simulink model "etasetget256Discretized2"  (R2015b)
settings: Solver=FixedStepAuto  StartTime=0.0  StopTime=inf  FixedStep=0.05  RelTol=1e-3
undefined symbols (not defined in the file or in its folder): X, Y, Z
libraries: robotlib x5
settings Model: Creator=einar  LastModifiedBy=einar
settings OptimizationCC: OptimizeModelRefInitCode=on  LifeSpan=Inf  MaxStackSize=64
settings HardwareCC: ProdBitPerPointer=32  ProdLargestAtomicFloat=None  ProdIntDivRoundTo=Undefined  ProdEndianess=Unspecified  ProdWordSize=32  ProdHWDeviceType=Generic->Unspecified (assume 32-bit Generic)
settings RTWCC: SystemTargetFile=ert.tlc  TemplateMakefile=ert_default_tmf  Description=Embedded Coder  Toolchain=Catkin  TargetLang=C++
settings CodeAppCC: IgnoreCustomStorageClasses=off
settings ERTTargetCC: SupportContinuousTime=on  SupportVariableSizeSignals=on

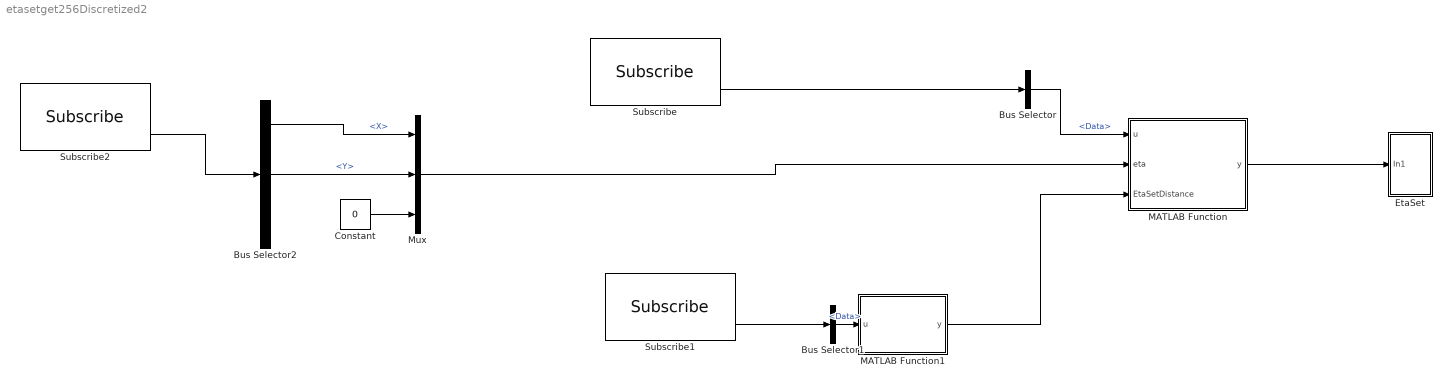
== system etasetget256Discretized2 ==
  Bus Selector : BusSelector  OutputSignals=Data
  Bus Selector1 : BusSelector  OutputSignals=Data
  Bus Selector2 : BusSelector  OutputSignals=X,Y,Z
  Constant : Constant  Value=0
  EtaSet : Subsystem
  MATLAB Function : MATLAB Function  TreatAsAtomicUnit=on
  MATLAB Function1 : MATLAB Function  TreatAsAtomicUnit=on
  Mux : Mux  Inputs=3
  Subscribe : robotlib/Subscribe  SourceLibraryInfo=This block requires Robotics System Toolbox  topicSource=Select from ROS network  topic=/EtaSetList  messageType=std_msgs/Float32MultiArray  sampleTime=-1  messageQueueLength=1
  Subscribe1 : robotlib/Subscribe  SourceLibraryInfo=This block requires Robotics System Toolbox  topicSource=Specify your own  topic=/EtaSetDistance  messageType=std_msgs/Float64  sampleTime=-1  messageQueueLength=1
  Subscribe2 : robotlib/Subscribe  SourceLibraryInfo=This block requires Robotics System Toolbox  topicSource=Specify your own  topic=/Eta  messageType=geometry_msgs/Vector3  sampleTime=-1  messageQueueLength=1
  wires:
  Subscribe/2 -> Bus Selector/1
  Bus Selector/1 -> MATLAB Function/1(u)  "<Data>"
  Mux/1 -> MATLAB Function/2(eta)
  MATLAB Function/1(y) -> EtaSet/1(In1)
  MATLAB Function1/1(y) -> MATLAB Function/3(EtaSetDistance)
  Subscribe1/2 -> Bus Selector1/1
  Bus Selector1/1 -> MATLAB Function1/1(u)  "<Data>"
  Bus Selector2/1 -> Mux/1  "<X>"
  Subscribe2/2 -> Bus Selector2/1
  Bus Selector2/2 -> Mux/2  "<Y>"
  Constant/1 -> Mux/3

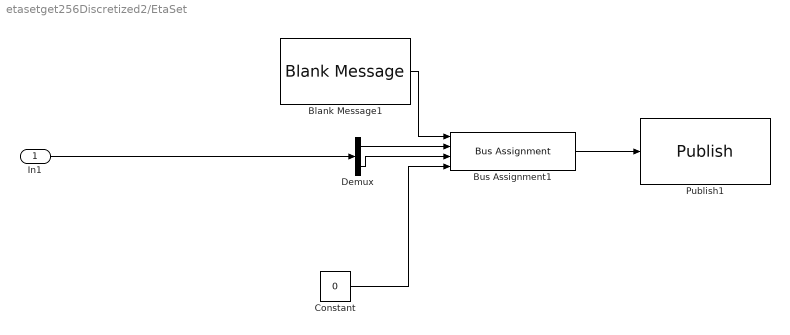
== system etasetget256Discretized2/EtaSet ==
  In1 : Inport
  Blank Message1 : robotlib/Blank Message  SourceLibraryInfo=This block requires Robotics System Toolbox  messageType=geometry_msgs/Vector3  SampleTime=inf
  Bus Assignment1 : BusAssignment  AssignedSignals=X,Y,Z
  Constant : Constant  Value=0
  Demux : Demux  Outputs=2
  Publish1 : robotlib/Publish  SourceLibraryInfo=This block requires Robotics System Toolbox  topicSource=Select from ROS network  topic=/EtaSet  messageType=geometry_msgs/Vector3  messageQueueLength=1
  wires:
  Bus Assignment1/1 -> Publish1/1
  Blank Message1/1 -> Bus Assignment1/1
  In1/1 -> Demux/1
  Demux/1 -> Bus Assignment1/2
  Demux/2 -> Bus Assignment1/3
  Constant/1 -> Bus Assignment1/4

== matlab function etasetget256Discretized2/MATLAB Function ==
  data: u input; y output; eta input; EtaSetDistance input
function y = fcn(u,eta,EtaSetDistance)

y=[0 0]
Z=length(u)
eta=eta(1:2);

%#codegen
%save('TESTlist2Eta')
Values=[u(1:Z/2) u(Z/2+1:end)];

Iterate2=min([find(Values==1000) ;size(Values,1)])

if u(1,1)==0&&sum((u==0))==Z;
    y=[0 0]
elseif Iterate2==2
%    asl=1
%    a=asl(2);
y(1)=Values(1,2)
y(2)=Values(1,1)
else
%DiscretizedPath
DiscretizedStep=0.01;
counter=1;
DiscretizedPath=zeros(5000,2);
for k=2:Iterate2-1
    DistanceTraveled=norm([Values(k,1)-Values(k-1,1) Values(k,2)-Values(k-1,2)]) ;
    DistanceTraveledX=Values(k,1)-Values(k-1,1);
    DistanceTraveledY=Values(k,2)-Values(k-1,2);
    Niterations=floor(DistanceTraveled/DiscretizedStep);
for z=1:Niterations
    DiscretizedPath(counter,1)=Values(k-1,1)+z*DistanceTraveledX/Niterations;
    DiscretizedPath(counter,2)=Values(k-1,2)+z*DistanceTraveledY/Niterations;
counter=counter+1;
end
end
DiscretizedEnds=min([find(DiscretizedPath==inf) ;size(DiscretizedPath,1)]);
DiscretizedPath=DiscretizedPath(1:DiscretizedEnds-1,1:2);

%%a=asl
eta=eta(2:-1:1)'

%Discretizing PathVector


NearestPointPos=4;
AvstandSaved=1000;
%for i=1:64
%AvstandDummy=(eta(1)-Values(i,1))^2+(eta(2)-Values(i,2))^2;
% if AvstandDummy<AvstandSaved
%     AvstandDummy=AvstandSaved;
% NearestPointPos=i;
% end
%end

    [Avstand NearestPointPos]=min((sum((abs(DiscretizedPath-repmat(eta,size(DiscretizedPath,1),1))).^2')));
if (NearestPointPos-3)>1
    SetPoint=NearestPointPos-3;

else SetPoint=1;
    
end
NIter=round(EtaSetDistance/DiscretizedStep);

SetPoint=max([1 NearestPointPos-NIter])
y(1)=DiscretizedPath(SetPoint,2)
y(2)=DiscretizedPath(SetPoint,1)
%etaset = u;11
%HEADING:
%end
end
y=y
end

== matlab function etasetget256Discretized2/MATLAB Function1 ==
  data: u input; y output
function y = fcn(u)

    y=u;    

if u==0
 y(1)=0.25
end
end
